simulink model "auto_linearize"  (R2020b)
settings: Solver=VariableStepAuto  StartTime=0.0  StopTime=10.0  RelTol=1e-3
values from neighbouring files (symbols this model uses):
  u1max = 25*pi/180    (= 0.436332312999)    [RCAM_initialization.m]
  u1min = -25*pi/180    (= -0.436332312999)    [RCAM_initialization.m]
  u2max = 10*pi/180    (= 0.174532925199)    [RCAM_initialization.m]
  u2min = -25*pi/180    (= -0.436332312999)    [RCAM_initialization.m]
  u3max = 30*pi/180    (= 0.523598775598)    [RCAM_initialization.m]
  u3min = -30*pi/180    (= -0.523598775598)    [RCAM_initialization.m]
  u4max = 10*pi/180    (= 0.174532925199)    [RCAM_initialization.m]
  u4min = 0.5*pi/180    (= 0.00872664625997)    [RCAM_initialization.m]
  u5max = 10*pi/180    (= 0.174532925199)    [RCAM_initialization.m]
  u5min = 0.5*pi/180    (= 0.00872664625997)    [RCAM_initialization.m]
  x0 = [85; 0; 0; 0; 0; 0; 0; 0; 0; xini; yini; h0]    [RCAM_initialization.m]
undefined symbols (not defined in the file or in its folder): RCAM_MODEL
settings Model: Creator=Yigit  LastModifiedBy=Yigit

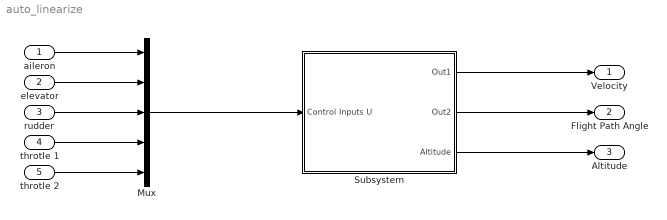
== system auto_linearize ==
  aileron : Inport
  elevator : Inport  Port=2
  rudder : Inport  Port=3
  throtle 1 : Inport  Port=4
  throtle 2 : Inport  Port=5
  Mux : Mux  Inputs=5
  Subsystem : Subsystem
  Velocity : Outport
  Flight Path Angle : Outport  Port=2
  Altitude : Outport  Port=3
  wires:
  aileron/1 -> Mux/1
  rudder/1 -> Mux/3
  throtle 1/1 -> Mux/4
  throtle 2/1 -> Mux/5
  elevator/1 -> Mux/2
  Mux/1 -> Subsystem/1(Control Inputs U)
  Subsystem/1(Out1) -> Velocity/1
  Subsystem/2(Out2) -> Flight Path Angle/1
  Subsystem/3(Altitude) -> Altitude/1

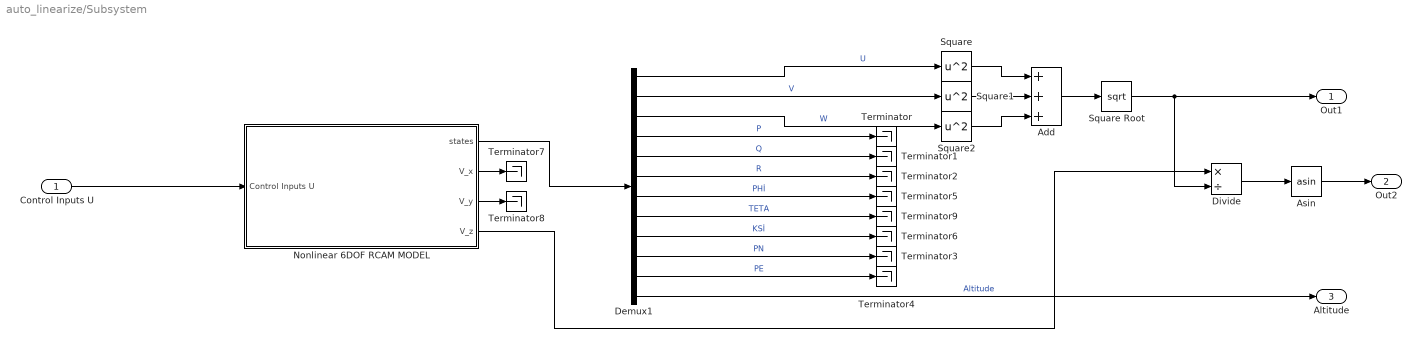
== system auto_linearize/Subsystem ==
  Control Inputs U : Inport
  Add : Sum  Inputs=+++
  Asin : Trigonometry  Operator=asin
  Demux1 : Demux  Outputs=12
  Divide : Product  Inputs=*/
  Nonlinear 6DOF RCAM MODEL : Subsystem
  Square : Math  Operator=square  SaturateOnIntegerOverflow=on
  Square Root : Sqrt  SaturateOnIntegerOverflow=on
  Square1 : Math  Operator=square  SaturateOnIntegerOverflow=on
  Square2 : Math  Operator=square  SaturateOnIntegerOverflow=on
  Terminator{,1..9} (10 alike) : Terminator
  Out1 : Outport
  Out2 : Outport  Port=2
  Altitude : Outport  Port=3
  wires:
  Square1/1 -> Add/2
  Demux1/1 -> Square/1  "U"
  Demux1/2 -> Square1/1  "V"
  Demux1/9 -> Terminator6/1  "KSİ"
  Square/1 -> Add/1
  Nonlinear 6DOF RCAM MODEL/1(states) -> Demux1/1
  Demux1/6 -> Terminator2/1  "R"
  Demux1/10 -> Terminator3/1  "PN"
  Demux1/11 -> Terminator4/1  "PE"
  Demux1/5 -> Terminator1/1  "Q"
  Demux1/4 -> Terminator/1  "P"
  Demux1/12 -> Altitude/1  "Altitude"
  Demux1/3 -> Square2/1  "W"
  Square2/1 -> Add/3
  Square Root/1 -> Divide/2, Out1/1
  Add/1 -> Square Root/1
  Demux1/7 -> Terminator5/1  "PHİ"
  Control Inputs U/1 -> Nonlinear 6DOF RCAM MODEL/1(Control Inputs U)
  Nonlinear 6DOF RCAM MODEL/2(V_x) -> Terminator7/1
  Nonlinear 6DOF RCAM MODEL/3(V_y) -> Terminator8/1
  Demux1/8 -> Terminator9/1  "TETA"
  Nonlinear 6DOF RCAM MODEL/4(V_z) -> Divide/1
  Divide/1 -> Asin/1
  Asin/1 -> Out2/1

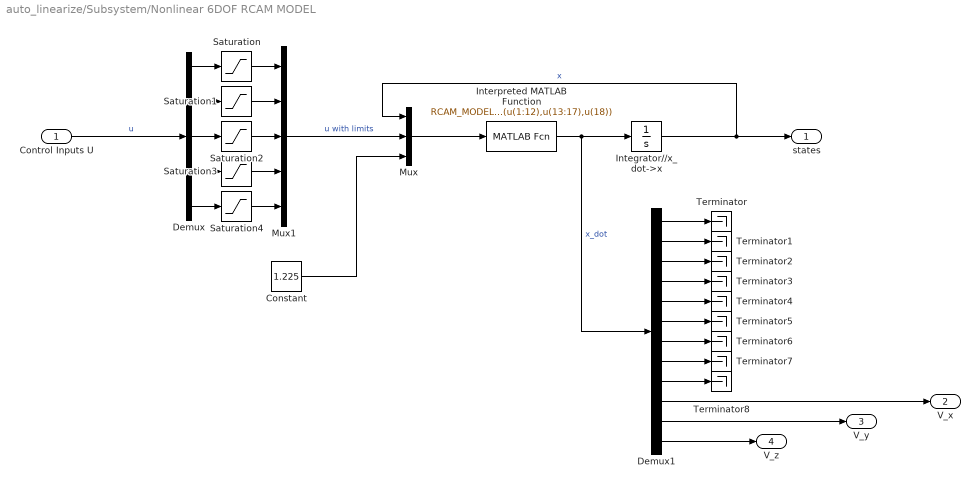
== system auto_linearize/Subsystem/Nonlinear 6DOF RCAM MODEL ==
  Control Inputs U : Inport
  Constant : Constant  Value=1.225
  Demux : Demux  Outputs=5
  Demux1 : Demux  Outputs=12
  Integrator//x_dot->x : Integrator  InitialCondition=x0
  Interpreted MATLAB Function : MATLABFcn  MATLABFcn=RCAM_MODEL(u(1:12),u(13:17),u(18))
  Mux : Mux  Inputs=3
  Mux1 : Mux  Inputs=5
  Saturation : Saturate  UpperLimit=u1max  LowerLimit=u1min
  Saturation1 : Saturate  UpperLimit=u2max  LowerLimit=u2min
  Saturation2 : Saturate  UpperLimit=u3max  LowerLimit=u3min
  Saturation3 : Saturate  UpperLimit=u4max  LowerLimit=u4min
  Saturation4 : Saturate  UpperLimit=u5max  LowerLimit=u5min
  Terminator{,1..8} (9 alike) : Terminator
  states : Outport
  V_x : Outport  Port=2
  V_y : Outport  Port=3
  V_z : Outport  Port=4
  wires:
  Interpreted MATLAB Function/1 -> Demux1/1, Integrator//x_dot->x/1  "x_dot"
  Mux/1 -> Interpreted MATLAB Function/1
  Integrator//x_dot->x/1 -> states/1, Mux/1  "x"
  Control Inputs U/1 -> Demux/1  "u"
  Demux/1 -> Saturation/1
  Demux/4 -> Saturation3/1
  Demux/5 -> Saturation4/1
  Demux/3 -> Saturation2/1
  Demux/2 -> Saturation1/1
  Saturation3/1 -> Mux1/4
  Saturation4/1 -> Mux1/5
  Saturation2/1 -> Mux1/3
  Saturation1/1 -> Mux1/2
  Saturation/1 -> Mux1/1
  Mux1/1 -> Mux/2  "u with limits"
  Constant/1 -> Mux/3
  Demux1/10 -> V_x/1
  Demux1/11 -> V_y/1
  Demux1/12 -> V_z/1
  Demux1/1 -> Terminator/1
  Demux1/2 -> Terminator1/1
  Demux1/3 -> Terminator2/1
  Demux1/4 -> Terminator3/1
  Demux1/5 -> Terminator4/1
  Demux1/6 -> Terminator5/1
  Demux1/7 -> Terminator6/1
  Demux1/8 -> Terminator7/1
  Demux1/9 -> Terminator8/1
